simulink model "Actormodel"  (R2018b)
(part 24 of 25)

  "IW{2,1}(433,:)'"/1 -> dotprod433/1
  dotprod433/1 -> Mux/433
  "IW{2,1}(434,:)'"/1 -> dotprod434/1
  dotprod434/1 -> Mux/434
  "IW{2,1}(435,:)'"/1 -> dotprod435/1
  dotprod435/1 -> Mux/435
  "IW{2,1}(436,:)'"/1 -> dotprod436/1
  dotprod436/1 -> Mux/436
  "IW{2,1}(437,:)'"/1 -> dotprod437/1
  dotprod437/1 -> Mux/437
  "IW{2,1}(438,:)'"/1 -> dotprod438/1
  dotprod438/1 -> Mux/438
  "IW{2,1}(439,:)'"/1 -> dotprod439/1
  dotprod439/1 -> Mux/439
  "IW{2,1}(440,:)'"/1 -> dotprod440/1
  dotprod440/1 -> Mux/440
  "IW{2,1}(441,:)'"/1 -> dotprod441/1
  dotprod441/1 -> Mux/441
  "IW{2,1}(442,:)'"/1 -> dotprod442/1
  dotprod442/1 -> Mux/442
  "IW{2,1}(443,:)'"/1 -> dotprod443/1
  dotprod443/1 -> Mux/443
  "IW{2,1}(444,:)'"/1 -> dotprod444/1
  dotprod444/1 -> Mux/444
  "IW{2,1}(445,:)'"/1 -> dotprod445/1
  dotprod445/1 -> Mux/445
  "IW{2,1}(446,:)'"/1 -> dotprod446/1
  dotprod446/1 -> Mux/446
  "IW{2,1}(447,:)'"/1 -> dotprod447/1
  dotprod447/1 -> Mux/447
  "IW{2,1}(448,:)'"/1 -> dotprod448/1
  dotprod448/1 -> Mux/448
  "IW{2,1}(449,:)'"/1 -> dotprod449/1
  dotprod449/1 -> Mux/449
  "IW{2,1}(450,:)'"/1 -> dotprod450/1
  dotprod450/1 -> Mux/450
  "IW{2,1}(451,:)'"/1 -> dotprod451/1
  dotprod451/1 -> Mux/451
  "IW{2,1}(452,:)'"/1 -> dotprod452/1
  dotprod452/1 -> Mux/452
  "IW{2,1}(453,:)'"/1 -> dotprod453/1
  dotprod453/1 -> Mux/453
  "IW{2,1}(454,:)'"/1 -> dotprod454/1
  dotprod454/1 -> Mux/454
  "IW{2,1}(455,:)'"/1 -> dotprod455/1
  dotprod455/1 -> Mux/455
  "IW{2,1}(456,:)'"/1 -> dotprod456/1
  dotprod456/1 -> Mux/456
  "IW{2,1}(457,:)'"/1 -> dotprod457/1
  dotprod457/1 -> Mux/457
  "IW{2,1}(458,:)'"/1 -> dotprod458/1
  dotprod458/1 -> Mux/458
  "IW{2,1}(459,:)'"/1 -> dotprod459/1
  dotprod459/1 -> Mux/459
  "IW{2,1}(460,:)'"/1 -> dotprod460/1
  dotprod460/1 -> Mux/460
  "IW{2,1}(461,:)'"/1 -> dotprod461/1
  dotprod461/1 -> Mux/461
  "IW{2,1}(462,:)'"/1 -> dotprod462/1
  dotprod462/1 -> Mux/462
  "IW{2,1}(463,:)'"/1 -> dotprod463/1
  dotprod463/1 -> Mux/463
  "IW{2,1}(464,:)'"/1 -> dotprod464/1
  dotprod464/1 -> Mux/464
  "IW{2,1}(465,:)'"/1 -> dotprod465/1
  dotprod465/1 -> Mux/465
  "IW{2,1}(466,:)'"/1 -> dotprod466/1
  dotprod466/1 -> Mux/466
  "IW{2,1}(467,:)'"/1 -> dotprod467/1
  dotprod467/1 -> Mux/467
  "IW{2,1}(468,:)'"/1 -> dotprod468/1
  dotprod468/1 -> Mux/468
  "IW{2,1}(469,:)'"/1 -> dotprod469/1
  dotprod469/1 -> Mux/469
  "IW{2,1}(470,:)'"/1 -> dotprod470/1
  dotprod470/1 -> Mux/470
  "IW{2,1}(471,:)'"/1 -> dotprod471/1
  dotprod471/1 -> Mux/471
  "IW{2,1}(472,:)'"/1 -> dotprod472/1
  dotprod472/1 -> Mux/472
  "IW{2,1}(473,:)'"/1 -> dotprod473/1
  dotprod473/1 -> Mux/473
  "IW{2,1}(474,:)'"/1 -> dotprod474/1
  dotprod474/1 -> Mux/474
  "IW{2,1}(475,:)'"/1 -> dotprod475/1
  dotprod475/1 -> Mux/475
  "IW{2,1}(476,:)'"/1 -> dotprod476/1
  dotprod476/1 -> Mux/476
  "IW{2,1}(477,:)'"/1 -> dotprod477/1
  dotprod477/1 -> Mux/477
  "IW{2,1}(478,:)'"/1 -> dotprod478/1
  dotprod478/1 -> Mux/478
  "IW{2,1}(479,:)'"/1 -> dotprod479/1
  dotprod479/1 -> Mux/479
  "IW{2,1}(480,:)'"/1 -> dotprod480/1
  dotprod480/1 -> Mux/480
  "IW{2,1}(481,:)'"/1 -> dotprod481/1
  dotprod481/1 -> Mux/481
  "IW{2,1}(482,:)'"/1 -> dotprod482/1
  dotprod482/1 -> Mux/482
  "IW{2,1}(483,:)'"/1 -> dotprod483/1
  dotprod483/1 -> Mux/483
  "IW{2,1}(484,:)'"/1 -> dotprod484/1
  dotprod484/1 -> Mux/484
  "IW{2,1}(485,:)'"/1 -> dotprod485/1
  dotprod485/1 -> Mux/485
  "IW{2,1}(486,:)'"/1 -> dotprod486/1
  dotprod486/1 -> Mux/486
  "IW{2,1}(487,:)'"/1 -> dotprod487/1
  dotprod487/1 -> Mux/487
  "IW{2,1}(488,:)'"/1 -> dotprod488/1
  dotprod488/1 -> Mux/488
  "IW{2,1}(489,:)'"/1 -> dotprod489/1
  dotprod489/1 -> Mux/489
  "IW{2,1}(490,:)'"/1 -> dotprod490/1
  dotprod490/1 -> Mux/490
  "IW{2,1}(491,:)'"/1 -> dotprod491/1
  dotprod491/1 -> Mux/491
  "IW{2,1}(492,:)'"/1 -> dotprod492/1
  dotprod492/1 -> Mux/492
  "IW{2,1}(493,:)'"/1 -> dotprod493/1
  dotprod493/1 -> Mux/493
  "IW{2,1}(494,:)'"/1 -> dotprod494/1
  dotprod494/1 -> Mux/494
  "IW{2,1}(495,:)'"/1 -> dotprod495/1
  dotprod495/1 -> Mux/495
  "IW{2,1}(496,:)'"/1 -> dotprod496/1
  dotprod496/1 -> Mux/496
  "IW{2,1}(497,:)'"/1 -> dotprod497/1
  dotprod497/1 -> Mux/497
  "IW{2,1}(498,:)'"/1 -> dotprod498/1
  dotprod498/1 -> Mux/498
  "IW{2,1}(499,:)'"/1 -> dotprod499/1
  dotprod499/1 -> Mux/499
  "IW{2,1}(500,:)'"/1 -> dotprod500/1
  dotprod500/1 -> Mux/500
  "IW{2,1}(501,:)'"/1 -> dotprod501/1
  dotprod501/1 -> Mux/501
  "IW{2,1}(502,:)'"/1 -> dotprod502/1
  dotprod502/1 -> Mux/502
  "IW{2,1}(503,:)'"/1 -> dotprod503/1
  dotprod503/1 -> Mux/503
  "IW{2,1}(504,:)'"/1 -> dotprod504/1
  dotprod504/1 -> Mux/504
  "IW{2,1}(505,:)'"/1 -> dotprod505/1
  dotprod505/1 -> Mux/505
  "IW{2,1}(506,:)'"/1 -> dotprod506/1
  dotprod506/1 -> Mux/506
  "IW{2,1}(507,:)'"/1 -> dotprod507/1
  dotprod507/1 -> Mux/507
  "IW{2,1}(508,:)'"/1 -> dotprod508/1
  dotprod508/1 -> Mux/508
  "IW{2,1}(509,:)'"/1 -> dotprod509/1
  dotprod509/1 -> Mux/509
  "IW{2,1}(510,:)'"/1 -> dotprod510/1
  dotprod510/1 -> Mux/510
  "IW{2,1}(511,:)'"/1 -> dotprod511/1
  dotprod511/1 -> Mux/511
  "IW{2,1}(512,:)'"/1 -> dotprod512/1
  dotprod512/1 -> Mux/512
  "IW{2,1}(513,:)'"/1 -> dotprod513/1
  dotprod513/1 -> Mux/513
  "IW{2,1}(514,:)'"/1 -> dotprod514/1
  dotprod514/1 -> Mux/514
  "IW{2,1}(515,:)'"/1 -> dotprod515/1
  dotprod515/1 -> Mux/515
  "IW{2,1}(516,:)'"/1 -> dotprod516/1
  dotprod516/1 -> Mux/516
  "IW{2,1}(517,:)'"/1 -> dotprod517/1
  dotprod517/1 -> Mux/517
  "IW{2,1}(518,:)'"/1 -> dotprod518/1
  dotprod518/1 -> Mux/518
  "IW{2,1}(519,:)'"/1 -> dotprod519/1
  dotprod519/1 -> Mux/519
  "IW{2,1}(520,:)'"/1 -> dotprod520/1
  dotprod520/1 -> Mux/520
  "IW{2,1}(521,:)'"/1 -> dotprod521/1
  dotprod521/1 -> Mux/521
  "IW{2,1}(522,:)'"/1 -> dotprod522/1
  dotprod522/1 -> Mux/522
  "IW{2,1}(523,:)'"/1 -> dotprod523/1
  dotprod523/1 -> Mux/523
  "IW{2,1}(524,:)'"/1 -> dotprod524/1
  dotprod524/1 -> Mux/524
  "IW{2,1}(525,:)'"/1 -> dotprod525/1
  dotprod525/1 -> Mux/525
  "IW{2,1}(526,:)'"/1 -> dotprod526/1
  dotprod526/1 -> Mux/526
  "IW{2,1}(527,:)'"/1 -> dotprod527/1
  dotprod527/1 -> Mux/527
  "IW{2,1}(528,:)'"/1 -> dotprod528/1
  dotprod528/1 -> Mux/528
  "IW{2,1}(529,:)'"/1 -> dotprod529/1
  dotprod529/1 -> Mux/529
  "IW{2,1}(530,:)'"/1 -> dotprod530/1
  dotprod530/1 -> Mux/530
  "IW{2,1}(531,:)'"/1 -> dotprod531/1
  dotprod531/1 -> Mux/531
  "IW{2,1}(532,:)'"/1 -> dotprod532/1
  dotprod532/1 -> Mux/532
  "IW{2,1}(533,:)'"/1 -> dotprod533/1
  dotprod533/1 -> Mux/533
  "IW{2,1}(534,:)'"/1 -> dotprod534/1
  dotprod534/1 -> Mux/534
  "IW{2,1}(535,:)'"/1 -> dotprod535/1
  dotprod535/1 -> Mux/535
  "IW{2,1}(536,:)'"/1 -> dotprod536/1
  dotprod536/1 -> Mux/536
  "IW{2,1}(537,:)'"/1 -> dotprod537/1
  dotprod537/1 -> Mux/537
  "IW{2,1}(538,:)'"/1 -> dotprod538/1
  dotprod538/1 -> Mux/538
  "IW{2,1}(539,:)'"/1 -> dotprod539/1
  dotprod539/1 -> Mux/539
  "IW{2,1}(540,:)'"/1 -> dotprod540/1
  dotprod540/1 -> Mux/540
  "IW{2,1}(541,:)'"/1 -> dotprod541/1
  dotprod541/1 -> Mux/541
  "IW{2,1}(542,:)'"/1 -> dotprod542/1
  dotprod542/1 -> Mux/542
  "IW{2,1}(543,:)'"/1 -> dotprod543/1
  dotprod543/1 -> Mux/543
  "IW{2,1}(544,:)'"/1 -> dotprod544/1
  dotprod544/1 -> Mux/544
  "IW{2,1}(545,:)'"/1 -> dotprod545/1
  dotprod545/1 -> Mux/545
  "IW{2,1}(546,:)'"/1 -> dotprod546/1
  dotprod546/1 -> Mux/546
  "IW{2,1}(547,:)'"/1 -> dotprod547/1
  dotprod547/1 -> Mux/547
  "IW{2,1}(548,:)'"/1 -> dotprod548/1
  dotprod548/1 -> Mux/548
  "IW{2,1}(549,:)'"/1 -> dotprod549/1
  dotprod549/1 -> Mux/549
  "IW{2,1}(550,:)'"/1 -> dotprod550/1
  dotprod550/1 -> Mux/550
  "IW{2,1}(551,:)'"/1 -> dotprod551/1
  dotprod551/1 -> Mux/551
  "IW{2,1}(552,:)'"/1 -> dotprod552/1
  dotprod552/1 -> Mux/552
  "IW{2,1}(553,:)'"/1 -> dotprod553/1
  dotprod553/1 -> Mux/553
  "IW{2,1}(554,:)'"/1 -> dotprod554/1
  dotprod554/1 -> Mux/554
  "IW{2,1}(555,:)'"/1 -> dotprod555/1
  dotprod555/1 -> Mux/555
  "IW{2,1}(556,:)'"/1 -> dotprod556/1
  dotprod556/1 -> Mux/556
  "IW{2,1}(557,:)'"/1 -> dotprod557/1
  dotprod557/1 -> Mux/557
  "IW{2,1}(558,:)'"/1 -> dotprod558/1
  dotprod558/1 -> Mux/558
  "IW{2,1}(559,:)'"/1 -> dotprod559/1
  dotprod559/1 -> Mux/559
  "IW{2,1}(560,:)'"/1 -> dotprod560/1
  dotprod560/1 -> Mux/560
  "IW{2,1}(561,:)'"/1 -> dotprod561/1
  dotprod561/1 -> Mux/561
  "IW{2,1}(562,:)'"/1 -> dotprod562/1
  dotprod562/1 -> Mux/562
  "IW{2,1}(563,:)'"/1 -> dotprod563/1
  dotprod563/1 -> Mux/563
  "IW{2,1}(564,:)'"/1 -> dotprod564/1
  dotprod564/1 -> Mux/564
  "IW{2,1}(565,:)'"/1 -> dotprod565/1
  dotprod565/1 -> Mux/565
  "IW{2,1}(566,:)'"/1 -> dotprod566/1
  dotprod566/1 -> Mux/566
  "IW{2,1}(567,:)'"/1 -> dotprod567/1
  dotprod567/1 -> Mux/567
  "IW{2,1}(568,:)'"/1 -> dotprod568/1
  dotprod568/1 -> Mux/568
  "IW{2,1}(569,:)'"/1 -> dotprod569/1
  dotprod569/1 -> Mux/569
  "IW{2,1}(570,:)'"/1 -> dotprod570/1
  dotprod570/1 -> Mux/570
  "IW{2,1}(571,:)'"/1 -> dotprod571/1
  dotprod571/1 -> Mux/571
  "IW{2,1}(572,:)'"/1 -> dotprod572/1
  dotprod572/1 -> Mux/572
  "IW{2,1}(573,:)'"/1 -> dotprod573/1
  dotprod573/1 -> Mux/573
  "IW{2,1}(574,:)'"/1 -> dotprod574/1
  dotprod574/1 -> Mux/574
  "IW{2,1}(575,:)'"/1 -> dotprod575/1
  dotprod575/1 -> Mux/575
  "IW{2,1}(576,:)'"/1 -> dotprod576/1
  dotprod576/1 -> Mux/576
  "IW{2,1}(577,:)'"/1 -> dotprod577/1
  dotprod577/1 -> Mux/577
  "IW{2,1}(578,:)'"/1 -> dotprod578/1
  dotprod578/1 -> Mux/578
  "IW{2,1}(579,:)'"/1 -> dotprod579/1
  dotprod579/1 -> Mux/579
  "IW{2,1}(580,:)'"/1 -> dotprod580/1
  dotprod580/1 -> Mux/580
  "IW{2,1}(581,:)'"/1 -> dotprod581/1
  dotprod581/1 -> Mux/581
  "IW{2,1}(582,:)'"/1 -> dotprod582/1
  dotprod582/1 -> Mux/582
  "IW{2,1}(583,:)'"/1 -> dotprod583/1
  dotprod583/1 -> Mux/583
  "IW{2,1}(584,:)'"/1 -> dotprod584/1
  dotprod584/1 -> Mux/584
  "IW{2,1}(585,:)'"/1 -> dotprod585/1
  dotprod585/1 -> Mux/585
  "IW{2,1}(586,:)'"/1 -> dotprod586/1
  dotprod586/1 -> Mux/586
  "IW{2,1}(587,:)'"/1 -> dotprod587/1
  dotprod587/1 -> Mux/587
  "IW{2,1}(588,:)'"/1 -> dotprod588/1
  dotprod588/1 -> Mux/588
  "IW{2,1}(589,:)'"/1 -> dotprod589/1
  dotprod589/1 -> Mux/589
  "IW{2,1}(590,:)'"/1 -> dotprod590/1
  dotprod590/1 -> Mux/590
  "IW{2,1}(591,:)'"/1 -> dotprod591/1
  dotprod591/1 -> Mux/591
  "IW{2,1}(592,:)'"/1 -> dotprod592/1
  dotprod592/1 -> Mux/592
  "IW{2,1}(593,:)'"/1 -> dotprod593/1
  dotprod593/1 -> Mux/593
  "IW{2,1}(594,:)'"/1 -> dotprod594/1
  dotprod594/1 -> Mux/594
  "IW{2,1}(595,:)'"/1 -> dotprod595/1
  dotprod595/1 -> Mux/595
  "IW{2,1}(596,:)'"/1 -> dotprod596/1
  dotprod596/1 -> Mux/596
  "IW{2,1}(597,:)'"/1 -> dotprod597/1
  dotprod597/1 -> Mux/597
  "IW{2,1}(598,:)'"/1 -> dotprod598/1
  dotprod598/1 -> Mux/598
  "IW{2,1}(599,:)'"/1 -> dotprod599/1
  dotprod599/1 -> Mux/599
  "IW{2,1}(600,:)'"/1 -> dotprod600/1
  dotprod600/1 -> Mux/600
  Mux/1 -> "lz{2,1}"/1
